simulink model "Closed_Loop"  (Simulink 7.9)
settings: Solver=ode45  StartTime=0.0  StopTime=1  RelTol=1e-3
libraries: powerlib x41, powerlib_extras x3
settings Model: Creator=Admin  LastModifiedBy=Admin

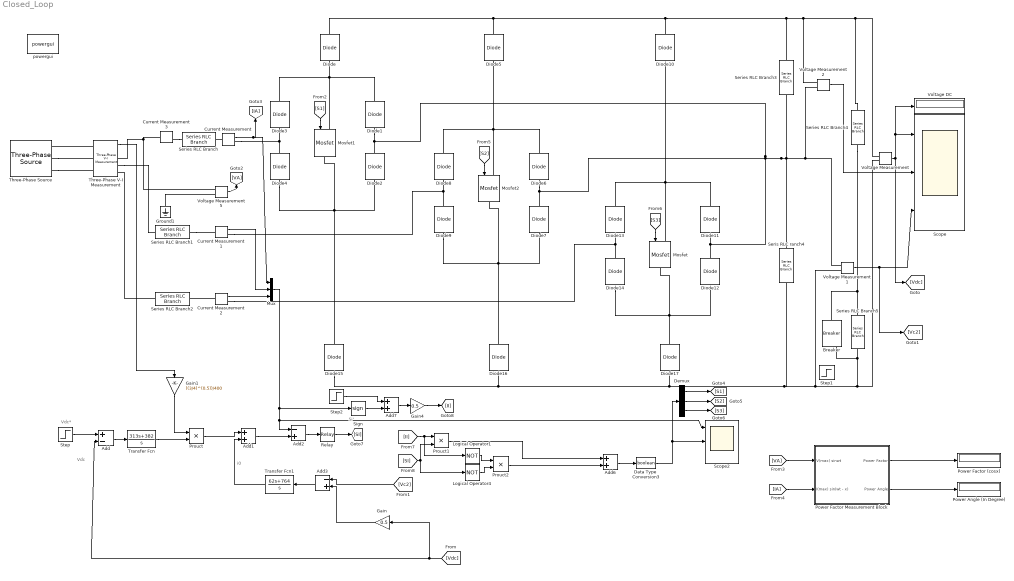
== system Closed_Loop ==
  note: Vdc
  note: Vdc*
  note: Si'
  note: i0
  Add : Sum  Inputs=+-
  Add1 : Sum
  Add2 : Sum  Inputs=-+
  Add3 : Sum  Inputs=-+
  Add6 : Sum
  Add7 : Sum
  Breaker : powerlib/Elements/Breaker  BreakerResistance=0.01  InitialState=0  SnubberResistance=1e6  SnubberCapacitance=inf  SwitchingTimes="[ 1/60  5/60 ]"  External=on  Measurements=None  MoreParameters=off  NoBreakLoop=off
  Current Measurement{,1..3} (4 alike) : powerlib/Measurements/Current Measurement  PhasorSimulation=off  OutputType=Complex  PSBequivalent=0
  Data Type  Conversion3 : DataTypeConversion  OutDataTypeStr=boolean  SaturateOnIntegerOverflow=on  RndMeth=Zero
  Demux : Demux  Outputs=3
  Diode{,1..17} (18 alike) : powerlib/Power Electronics/Diode  Ron=0.001  Lon=0  Vf=0.8  IC=0  UseSnubber=off  Rs=500  Cs=250e-9  Measurements=off
  Gain : Gain  Gain=0.5
  Gain1 : Gain  Gain=((3/4)^(0.5))/400
  Gain4 : Gain  Gain=0.5
  Ground1 : powerlib/Elements/Ground  LConnTagsString=a
  Logical Operator1 : Logic  Operator=NOT  AllPortsSameDT=off  OutDataTypeStr=boolean
  Logical Operator4 : Logic  Operator=NOT  AllPortsSameDT=off  OutDataTypeStr=boolean
  Mosfet : powerlib/Power Electronics/Mosfet  Ron=0.1  Lon=0  Rd=0.01  Vfd=0  IC=0  Rs=1e5  Cs=inf  Measurements=off
  Mosfet1 : powerlib/Power Electronics/Mosfet  Ron=0.1  Lon=0  Rd=0.01  Vfd=0  IC=0  Rs=1e5  Cs=inf  Measurements=off
  Mosfet2 : powerlib/Power Electronics/Mosfet  Ron=0.1  Lon=0  Rd=0.01  Vfd=0  IC=0  Rs=1e5  Cs=inf  Measurements=off
  Mux : Mux  Inputs=3
  Power Angle (In Degree) : Display
  Power Factor (cosx) : Display
  Power Factor Measurement Block : Subsystem  RequirementInfo={} %GIDa_9d9cfc83_43cf_4ce7_b51e_2d10133dbc8d
  Prouct : Product  RndMeth=Zero
  Prouct1 : Product  RndMeth=Zero
  Prouct2 : Product  RndMeth=Zero
  Relay : Relay  OnSwitchValue=0.01  OffSwitchValue=-0.01
  Scope : Scope  NumInputPorts=3
      settings: TimeRange=0.4  YMin=762.5~445~315  YMax=800~475~326  SaveName=Vdc
  Scope2 : Scope  NumInputPorts=3
      settings: YMin=-125~-0.1~-100000  YMax=150~1~100000  SaveName=Isbc1
  Series RLC Branch : powerlib/Elements/Series RLC Branch  LConnTagsString=__new0  RConnTagsString=__new0  BranchType=L  Resistance=1  Inductance=20e-3  SetiL0=off  InitialCurrent=0  Capacitance=1e-6  Setx0=off  InitialVoltage=0  Measurements=None
  Series RLC Branch1 : powerlib/Elements/Series RLC Branch  LConnTagsString=__new0  RConnTagsString=__new0  BranchType=L  Resistance=1  Inductance=20e-3  SetiL0=off  InitialCurrent=0  Capacitance=1e-6  Setx0=off  InitialVoltage=0  Measurements=None
  Series RLC Branch2 : powerlib/Elements/Series RLC Branch  LConnTagsString=__new0  RConnTagsString=__new0  BranchType=L  Resistance=1  Inductance=20e-3  SetiL0=off  InitialCurrent=0  Capacitance=1e-6  Setx0=off  InitialVoltage=0  Measurements=None
  Series RLC Branch3 : powerlib/Elements/Series RLC Branch  LConnTagsString=__new0  RConnTagsString=__new0  BranchType=C  Resistance=1  Inductance=1e-3  SetiL0=off  InitialCurrent=0  Capacitance=470e-6  Setx0=off  InitialVoltage=0  Measurements=None
  Series RLC Branch4 : powerlib/Elements/Series RLC Branch  LConnTagsString=__new0  RConnTagsString=__new0  BranchType=R  Resistance=200  Inductance=1e-3  SetiL0=off  InitialCurrent=0  Capacitance=1e-6  Setx0=off  InitialVoltage=0  Measurements=None
  Series RLC Branch5 : powerlib/Elements/Series RLC Branch  LConnTagsString=__new0  RConnTagsString=__new0  BranchType=R  Resistance=200  Inductance=1e-3  SetiL0=off  InitialCurrent=0  Capacitance=1e-6  Setx0=off  InitialVoltage=0  Measurements=None
  Seris RLC ranch4 : powerlib/Elements/Series RLC Branch  LConnTagsString=__new0  RConnTagsString=__new0  BranchType=C  Resistance=1  Inductance=1e-3  SetiL0=off  InitialCurrent=0  Capacitance=470e-6  Setx0=off  InitialVoltage=0  Measurements=None
  Sign : Signum
  Step : Step  Time=0  Before=750  After=750  SampleTime=0  VectorParams1D=off
  Step1 : Step  Time=0.2  SampleTime=0
  Step2 : Step  Time=0  Before=1  SampleTime=0  VectorParams1D=off
  Three-Phase V-I Measurement : powerlib/Measurements/Three-Phase V-I Measurement  VoltageMeasurement=phase-to-ground  SetLabelV=off  LabelV=Vabc  Vpu=off  VpuLL=off  CurrentMeasurement=yes  SetLabelI=off  LabelI=Iabc  Ipu=off  Pbase=100e6  Vbase=500e3  OutputType=Complex  PhasorSimulation=off  PSBequivalent=0
  Three-Phase Source : powerlib/Electrical Sources/Three-Phase Source  Voltage=400*(2^(0.5))  PhaseAngle=0  Frequency=50  InternalConnection=Yg  SpecifyImpedance=off  Resistance=0  Inductance=0  ShortCircuitLevel=100e6  BaseVoltage=25e3  XRratio=7  BusType=swing  Pref=0  Qref=0  Qmin=-inf  Qmax=inf
  Transfer Fcn : TransferFcn  Numerator=[313 382]  Denominator=[1 0]
  Transfer Fcn1 : TransferFcn  Numerator=[62 764]  Denominator=[1 0]
  Voltage DC : Display
  Voltage Measurement{,1..2,5} (4 alike) : powerlib/Measurements/Voltage Measurement  PhasorSimulation=off  OutputType=Complex  PSBequivalent=0
  powergui : powerlib/powergui  Priority=1  SimulationMode=Discrete  SolverType=Tustin  SampleTime=1/20000  frequency=60  SPID=off  DisableSnubberDevices=on  DisableRonSwitches=on  DisableVfSwitches=on  SwTol=0  Interpol=off  DisplayEquations=off  FunctionMessages=off  frequencyindice=50  Pbase=100e6  ErrMax=1e-4  Iterations=50  UnitsV=kV  UnitsW=MW  echomessages=off  HookPort=off  EnableUseOfTLC=off  x0status=blocks  RestoreLinks=warning  ResistiveCurrentMeasurement=off  Ylog=off  Xlog=on  ShowGrid=off  save=off  variable=ZData  structure=Isbc1  ZoomFFT=off  StartTime=0.8  cycles=2  DisplayStyle=1  fundamental=50  FreqAxis=off  MaxFrequency=1000  frequencyindicesteady=1  display=off  methode=off
  wires:
  Voltage Measurement/1 -> [Vdc], Scope/1, Voltage DC/1
  Step/1 -> Add/1
  Add/1 -> Transfer Fcn/1
  Transfer Fcn/1 -> Prouct/2
  Prouct/1 -> Add1/1
  Add1/1 -> Add2/2
  Add2/1 -> Relay/1
  Gain/1 -> Add3/2
  [Vdc] -> Gain/1, Add/2
  Voltage Measurement1/1 -> [Vc2], Scope/3
  [Vc2] -> Add3/1
  Gain1/1 -> Prouct/1
  Three-Phase V-I Measurement/1 -> Gain1/1
  Current Measurement2/1 -> Mux/3
  Current Measurement1/1 -> Mux/2
  Current Measurement/1 -> Mux/1, [IA]
  Mux/1 -> Sign/1, Add2/1, Scope2/1
  Voltage Measurement2/1 -> Scope/2
  Power Factor Measurement Block/1(Power Factor) -> Power Factor (cosx)/1
  Power Factor Measurement Block/2(Power Angle) -> Power Angle (In Degree)/1
  Voltage Measurement5/1 -> [VA]
  Demux/1 -> [S1]
  Demux/2 -> [S2]
  Demux/3 -> [S3]
  [S1] -> Mosfet1/1
  [S2] -> Mosfet2/1
  [S3] -> Mosfet/1
  [VA] -> Power Factor Measurement Block/1(V(max) sinwt)
  [IA] -> Power Factor Measurement Block/2(I(max) sin(wt - x))
  Transfer Fcn1/1 -> Add1/2
  Add3/1 -> Transfer Fcn1/1
  [SI] -> Prouct1/2, Logical Operator4/1
  Sign/1 -> Add7/2
  Step2/1 -> Add7/1
  Add7/1 -> Gain4/1
  Gain4/1 -> [II]
  [II] -> Prouct1/1, Logical Operator1/1
  Prouct1/1 -> Add6/1
  Logical Operator1/1 -> Prouct2/1
  Logical Operator4/1 -> Prouct2/2
  Prouct2/1 -> Add6/2
  Add6/1 -> Data Type  Conversion3/1
  Data Type  Conversion3/1 -> Scope2/2, Demux/1
  Relay/1 -> [SI]
  connections:
  Diode4/RConn1 -- Diode3/LConn1 -- Current Measurement/RConn1
  Mosfet1/LConn1 -- Diode/LConn1 -- Diode3/RConn1 -- Diode1/RConn1
  Mosfet1/RConn1 -- Diode4/LConn1 -- Diode2/LConn1 -- Diode15/RConn1
  Mosfet2/LConn1 -- Diode6/RConn1 -- Diode5/LConn1 -- Diode8/RConn1
  Mosfet2/RConn1 -- Diode9/LConn1 -- Diode7/LConn1 -- Diode16/RConn1
  Diode9/RConn1 -- Diode8/LConn1 -- Current Measurement1/RConn1
  Mosfet/LConn1 -- Diode11/RConn1 -- Diode10/LConn1 -- Diode13/RConn1
  Mosfet/RConn1 -- Diode14/LConn1 -- Diode12/LConn1 -- Diode17/RConn1
  Diode14/RConn1 -- Diode13/LConn1 -- Current Measurement2/RConn1
  Diode15/LConn1 -- Diode16/LConn1 -- Diode17/LConn1 -- Seris RLC ranch4/RConn1 -- Voltage Measurement1/LConn2 -- Voltage Measurement/LConn2 -- Series RLC Branch5/RConn1 -- Breaker/LConn1
  Series RLC Branch4/LConn1 -- Diode/RConn1 -- Diode5/RConn1 -- Diode10/RConn1 -- Series RLC Branch3/LConn1 -- Voltage Measurement2/LConn1 -- Voltage Measurement/LConn1
  Series RLC Branch2/LConn1 -- Three-Phase V-I Measurement/RConn3
  Voltage Measurement5/LConn1 -- Three-Phase V-I Measurement/RConn1 -- Current Measurement3/LConn1
  Three-Phase V-I Measurement/RConn2 -- Series RLC Branch1/LConn1
  Three-Phase V-I Measurement/LConn1 -- Three-Phase Source/RConn1
  Three-Phase Source/RConn2 -- Three-Phase V-I Measurement/LConn2
  Three-Phase Source/RConn3 -- Three-Phase V-I Measurement/LConn3
  Voltage Measurement1/LConn1 -- Diode6/LConn1 -- Diode7/RConn1 -- Diode1/LConn1 -- Diode2/RConn1 -- Diode12/RConn1 -- Diode11/LConn1 -- Series RLC Branch3/RConn1 -- Seris RLC ranch4/LConn1 -- Voltage Measurement2/LConn2
  Current Measurement2/LConn1 -- Series RLC Branch2/RConn1
  Series RLC Branch1/RConn1 -- Current Measurement1/LConn1
  Current Measurement/LConn1 -- Series RLC Branch/RConn1
  Series RLC Branch4/RConn1 -- Series RLC Branch5/LConn1 -- Breaker/RConn1
  Voltage Measurement5/LConn2 -- Ground1/LConn1
  Current Measurement3/RConn1 -- Series RLC Branch/LConn1

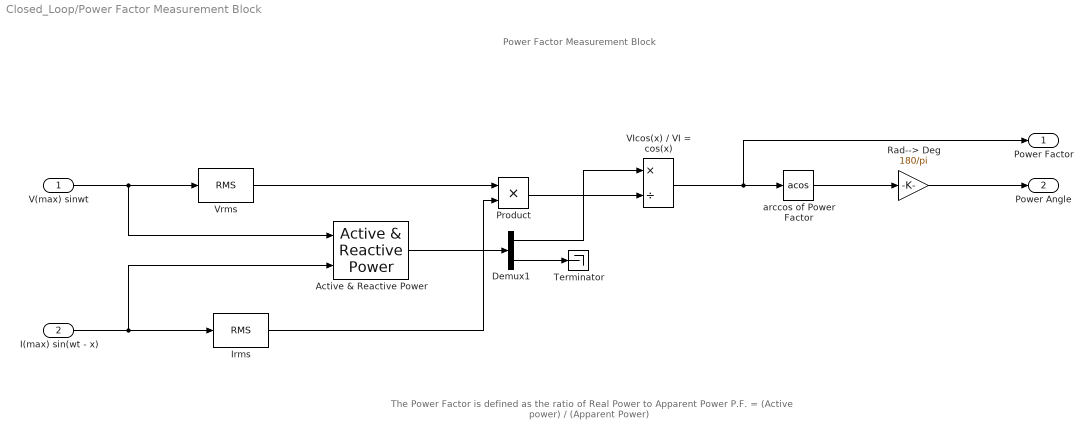
== system Closed_Loop/Power Factor Measurement Block ==
  note: The Power Factor is defined as the ratio of Real Power to Apparent Power
      | P.F. = (Active power) / (Apparent Power)
  note: Power Factor Measurement Block
  V(max) sinwt : Inport
  I(max) sin(wt - x) : Inport  Port=2
  Active & Reactive Power : powerlib_extras/Measurements/Active & Reactive Power  f1=50
  Demux1 : Demux  Outputs=2
  Irms : powerlib_extras/Measurements/RMS  f1=50
  Product : Product  RndMeth=Zero
  Rad--> Deg : Gain  Gain=180/pi  SaturateOnIntegerOverflow=on  OutDataTypeStr=Inherit: Same as input  ParamDataTypeStr=Inherit: Same as input
  Terminator : Terminator
  VIcos(x) / VI = cos(x) : Product  Inputs=*/
  Vrms : powerlib_extras/Measurements/RMS  f1=50
  arccos of Power Factor : Trigonometry  Operator=acos  OutputSignalType=real
  Power Factor : Outport
  Power Angle : Outport  Port=2
  wires:
  Active & Reactive Power/1 -> Demux1/1
  Demux1/1 -> VIcos(x) / VI = cos(x)/1
  Vrms/1 -> Product/1
  Irms/1 -> Product/2
  Product/1 -> VIcos(x) / VI = cos(x)/2
  VIcos(x) / VI = cos(x)/1 -> arccos of Power Factor/1, Power Factor/1
  arccos of Power Factor/1 -> Rad--> Deg/1
  Rad--> Deg/1 -> Power Angle/1
  V(max) sinwt/1 -> Vrms/1, Active & Reactive Power/1
  I(max) sin(wt - x)/1 -> Irms/1, Active & Reactive Power/2
  Demux1/2 -> Terminator/1
